simulink model "windTurbineSimulation"  (R2022a)
settings: Solver=FixedStepAuto  StartTime=0.0  StopTime=1000  FixedStep=0.001  RelTol=1e-3
libraries: embmathops x3
settings Model: Creator=S3945888  LastModifiedBy=119617
settings DebuggingCC: UnconnectedInputMsg=warning  UnconnectedOutputMsg=warning  UnconnectedLineMsg=warning
settings RTWCC: DLArmComputeVersion=19.05

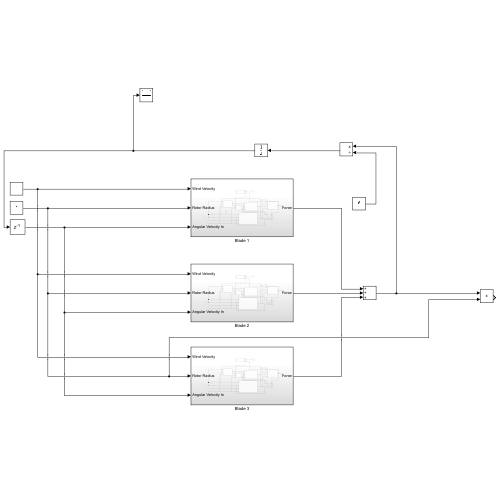
[thumbnail: Simulink's stored preview of the top-level diagram]
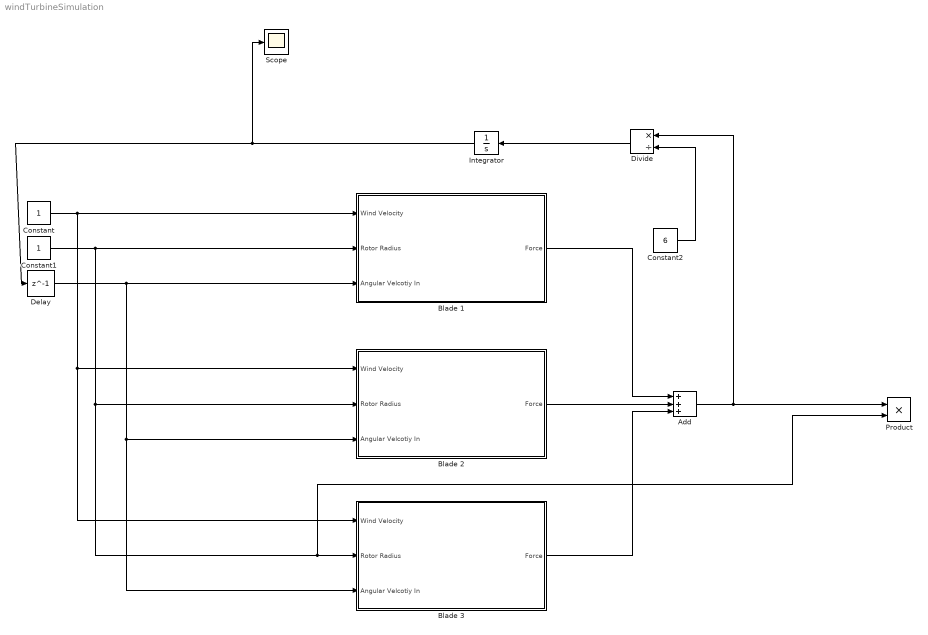
== system windTurbineSimulation ==
  Add : Sum  Inputs=+++
  Blade 1 : Subsystem
  Blade 2 : Subsystem
  Blade 3 : Subsystem
  Constant : Constant
  Constant1 : Constant
  Constant2 : Constant  Value=6
  Delay : Delay  DelayLength=1  InitialCondition=-6
  Divide : Product  Inputs=*/
  Integrator : Integrator  InitialCondition=-6
  Product : Product
  Scope : Scope
  wires:
  Constant/1 -> Blade 3/1(Wind Velocity), Blade 2/1(Wind Velocity), Blade 1/1(Wind Velocity)
  Constant1/1 -> Product/2, Blade 3/2(Rotor Radius), Blade 2/2(Rotor Radius), Blade 1/2(Rotor Radius)
  Blade 1/1(Force) -> Add/1
  Blade 2/1(Force) -> Add/2
  Blade 3/1(Force) -> Add/3
  Add/1 -> Divide/1, Product/1
  Delay/1 -> Blade 1/3(Angular Velcotiy In), Blade 3/3(Angular Velcotiy In), Blade 2/3(Angular Velcotiy In)
  Constant2/1 -> Divide/2
  Divide/1 -> Integrator/1
  Integrator/1 -> Scope/1, Delay/1

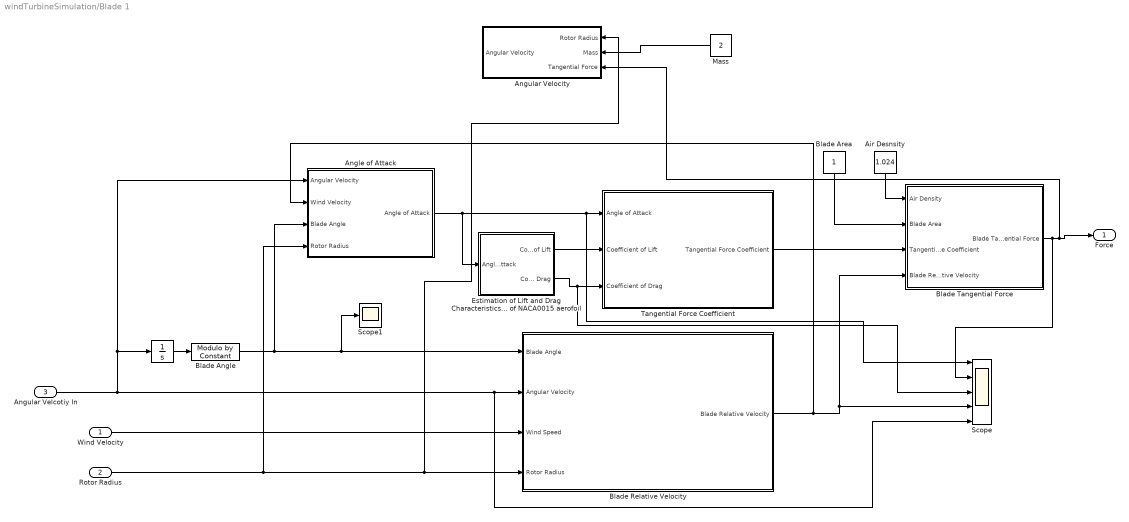
== system windTurbineSimulation/Blade 1 ==
  Wind Velocity : Inport
  Rotor Radius : Inport  Port=2
  Angular Velcotiy In : Inport  Port=3
  " " : Integrator
  Air Desnsity : Constant  Value=1.024
  Angle of Attack : Subsystem
  Angular Velocity : Subsystem
  Blade Angle : embmathops/Modulo by Constant  Denominator=2*pi  SimulateUsing=Code generation
      settings: SourceProductBaseCode=SL
  Blade Area : Constant
  Blade Relative Velocity : Subsystem
  Blade Tangential Force : Subsystem
  Estimation of Lift and Drag Characteristics of NACA0015 aerofoil : Subsystem
  Mass : Constant  Value=2
  Scope : Scope  NumInputPorts=5
  Scope1 : Scope
  Tangential Force Coefficient : Subsystem
  Force : Outport
  wires:
  Angular Velcotiy In/1 -> Angle of Attack/1(Angular Velocity), " "/1, Scope/5, Blade Relative Velocity/2(Angular Velocity)
  Air Desnsity/1 -> Blade Tangential Force/1(Air Density)
  Estimation of Lift and Drag Characteristics of NACA0015 aerofoil/2(Coefficient of Drag) -> Scope/3, Tangential Force Coefficient/3(Coefficient of Drag)
  Blade Angle/1 -> Angle of Attack/3(Blade Angle), Scope1/1, Blade Relative Velocity/1(Blade Angle)
  Tangential Force Coefficient/1(Tangential Force Coefficient) -> Blade Tangential Force/3(Tangential Force Coefficient)
  Angle of Attack/1(Angle of Attack) -> Scope/1, Tangential Force Coefficient/1(Angle of Attack), Estimation of Lift and Drag Characteristics of NACA0015 aerofoil/1(Angle of Attack)
  Blade Relative Velocity/1(Blade Relative Velocity) -> Angle of Attack/2(Wind Velocity), Scope/4, Blade Tangential Force/4(Blade Relative Velocity)
  Wind Velocity/1 -> Blade Relative Velocity/3(Wind Speed)
  Blade Tangential Force/1(Blade Tangential Force) -> Scope/2, Force/1, Angular Velocity/3(Tangential Force)
  Estimation of Lift and Drag Characteristics of NACA0015 aerofoil/1(Coefficient of Lift) -> Tangential Force Coefficient/2(Coefficient of Lift)
  Blade Area/1 -> Blade Tangential Force/2("Blade Area ")
  Mass/1 -> Angular Velocity/2(Mass)
  Rotor Radius/1 -> Angle of Attack/4(Rotor Radius), Angular Velocity/1(Rotor Radius), Blade Relative Velocity/4(Rotor Radius)
  " "/1 -> Blade Angle/1

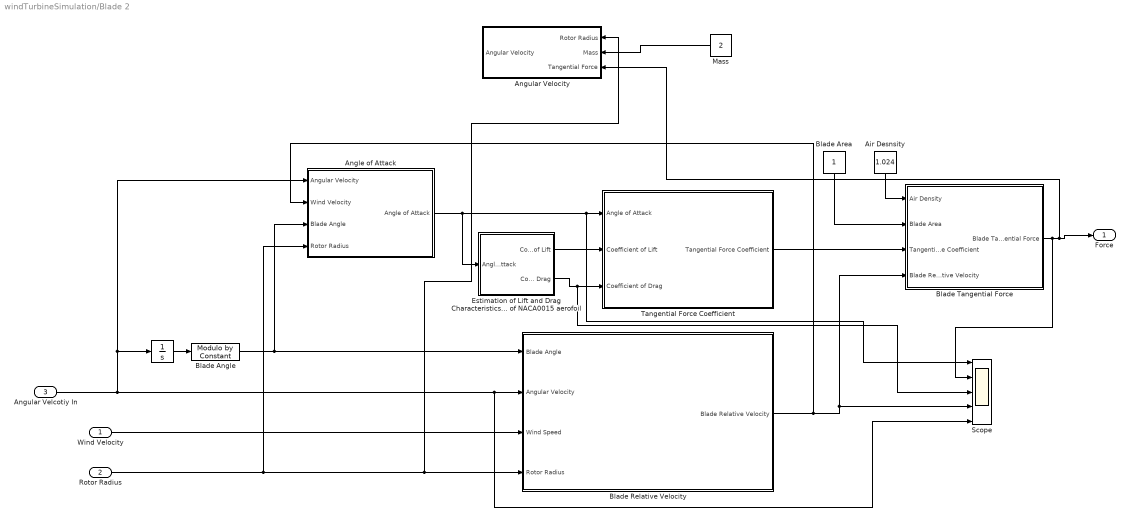
== system windTurbineSimulation/Blade 2 ==
  Wind Velocity : Inport
  Rotor Radius : Inport  Port=2
  Angular Velcotiy In : Inport  Port=3
  " " : Integrator
  Air Desnsity : Constant  Value=1.024
  Angle of Attack : Subsystem
  Angular Velocity : Subsystem
  Blade Angle : embmathops/Modulo by Constant  Denominator=2*pi  SimulateUsing=Code generation
      settings: SourceProductBaseCode=SL
  Blade Area : Constant
  Blade Relative Velocity : Subsystem
  Blade Tangential Force : Subsystem
  Estimation of Lift and Drag Characteristics of NACA0015 aerofoil : Subsystem
  Mass : Constant  Value=2
  Scope : Scope  NumInputPorts=5
  Tangential Force Coefficient : Subsystem
  Force : Outport
  wires:
  Angular Velcotiy In/1 -> Angle of Attack/1(Angular Velocity), " "/1, Scope/5, Blade Relative Velocity/2(Angular Velocity)
  Air Desnsity/1 -> Blade Tangential Force/1(Air Density)
  Estimation of Lift and Drag Characteristics of NACA0015 aerofoil/2(Coefficient of Drag) -> Scope/3, Tangential Force Coefficient/3(Coefficient of Drag)
  Blade Angle/1 -> Angle of Attack/3(Blade Angle), Blade Relative Velocity/1(Blade Angle)
  Tangential Force Coefficient/1(Tangential Force Coefficient) -> Blade Tangential Force/3(Tangential Force Coefficient)
  Angle of Attack/1(Angle of Attack) -> Scope/1, Tangential Force Coefficient/1(Angle of Attack), Estimation of Lift and Drag Characteristics of NACA0015 aerofoil/1(Angle of Attack)
  Blade Relative Velocity/1(Blade Relative Velocity) -> Angle of Attack/2(Wind Velocity), Scope/4, Blade Tangential Force/4(Blade Relative Velocity)
  Wind Velocity/1 -> Blade Relative Velocity/3(Wind Speed)
  Blade Tangential Force/1(Blade Tangential Force) -> Scope/2, Force/1, Angular Velocity/3(Tangential Force)
  Estimation of Lift and Drag Characteristics of NACA0015 aerofoil/1(Coefficient of Lift) -> Tangential Force Coefficient/2(Coefficient of Lift)
  Blade Area/1 -> Blade Tangential Force/2("Blade Area ")
  Mass/1 -> Angular Velocity/2(Mass)
  Rotor Radius/1 -> Angle of Attack/4(Rotor Radius), Angular Velocity/1(Rotor Radius), Blade Relative Velocity/4(Rotor Radius)
  " "/1 -> Blade Angle/1

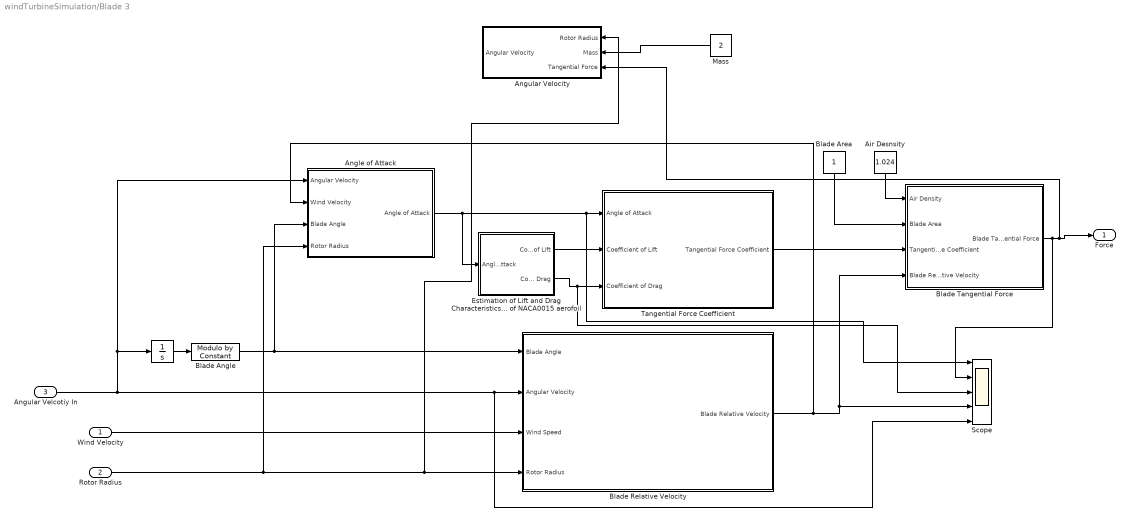
== system windTurbineSimulation/Blade 3 ==
  Wind Velocity : Inport
  Rotor Radius : Inport  Port=2
  Angular Velcotiy In : Inport  Port=3
  " " : Integrator
  Air Desnsity : Constant  Value=1.024
  Angle of Attack : Subsystem
  Angular Velocity : Subsystem
  Blade Angle : embmathops/Modulo by Constant  Denominator=2*pi  SimulateUsing=Code generation
      settings: SourceProductBaseCode=SL
  Blade Area : Constant
  Blade Relative Velocity : Subsystem
  Blade Tangential Force : Subsystem
  Estimation of Lift and Drag Characteristics of NACA0015 aerofoil : Subsystem
  Mass : Constant  Value=2
  Scope : Scope  NumInputPorts=5
  Tangential Force Coefficient : Subsystem
  Force : Outport
  wires:
  Angular Velcotiy In/1 -> Angle of Attack/1(Angular Velocity), " "/1, Scope/5, Blade Relative Velocity/2(Angular Velocity)
  Air Desnsity/1 -> Blade Tangential Force/1(Air Density)
  Estimation of Lift and Drag Characteristics of NACA0015 aerofoil/2(Coefficient of Drag) -> Scope/3, Tangential Force Coefficient/3(Coefficient of Drag)
  Blade Angle/1 -> Angle of Attack/3(Blade Angle), Blade Relative Velocity/1(Blade Angle)
  Tangential Force Coefficient/1(Tangential Force Coefficient) -> Blade Tangential Force/3(Tangential Force Coefficient)
  Angle of Attack/1(Angle of Attack) -> Scope/1, Tangential Force Coefficient/1(Angle of Attack), Estimation of Lift and Drag Characteristics of NACA0015 aerofoil/1(Angle of Attack)
  Blade Relative Velocity/1(Blade Relative Velocity) -> Angle of Attack/2(Wind Velocity), Scope/4, Blade Tangential Force/4(Blade Relative Velocity)
  Wind Velocity/1 -> Blade Relative Velocity/3(Wind Speed)
  Blade Tangential Force/1(Blade Tangential Force) -> Scope/2, Force/1, Angular Velocity/3(Tangential Force)
  Estimation of Lift and Drag Characteristics of NACA0015 aerofoil/1(Coefficient of Lift) -> Tangential Force Coefficient/2(Coefficient of Lift)
  Blade Area/1 -> Blade Tangential Force/2("Blade Area ")
  Mass/1 -> Angular Velocity/2(Mass)
  Rotor Radius/1 -> Angle of Attack/4(Rotor Radius), Angular Velocity/1(Rotor Radius), Blade Relative Velocity/4(Rotor Radius)
  " "/1 -> Blade Angle/1

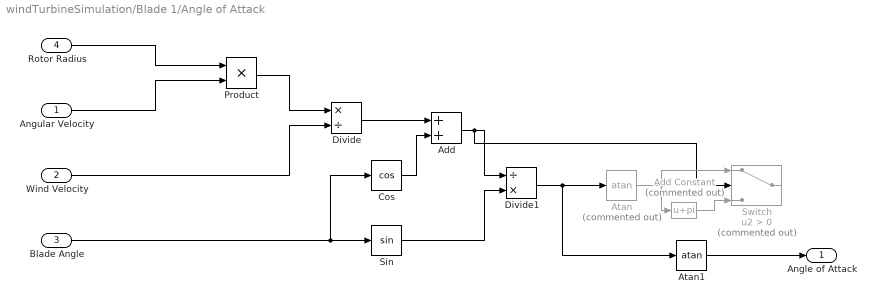
== system windTurbineSimulation/Blade 1/Angle of Attack ==
  Angular Velocity : Inport
  Wind Velocity : Inport  Port=2
  Blade Angle : Inport  Port=3
  Rotor Radius : Inport  Port=4
  Add : Sum
  Add Constant : Bias  Commented=on  Bias=pi  SaturateOnIntegerOverflow=off
  Atan : Trigonometry  Commented=on  Operator=atan
  Atan1 : Trigonometry  Operator=atan
  Cos : Trigonometry  Operator=cos
  Divide : Product  Inputs=*/
  Divide1 : Product  Inputs=/*
  Product : Product
  Sin : Trigonometry
  Switch : Switch  Commented=on  Criteria=u2 > Threshold  SaturateOnIntegerOverflow=off  InputSameDT=off
  Angle of Attack : Outport
  wires:
  Angular Velocity/1 -> Product/2
  Rotor Radius/1 -> Product/1
  Wind Velocity/1 -> Divide/2
  Product/1 -> Divide/1
  Divide/1 -> Add/1
  Cos/1 -> Add/2
  Blade Angle/1 -> Sin/1, Cos/1
  Add/1 -> Switch/2, Divide1/1
  Sin/1 -> Divide1/2
  Divide1/1 -> Atan1/1, Atan/1
  Atan/1 -> Add Constant/1, Switch/1
  Add Constant/1 -> Switch/3
  Atan1/1 -> Angle of Attack/1

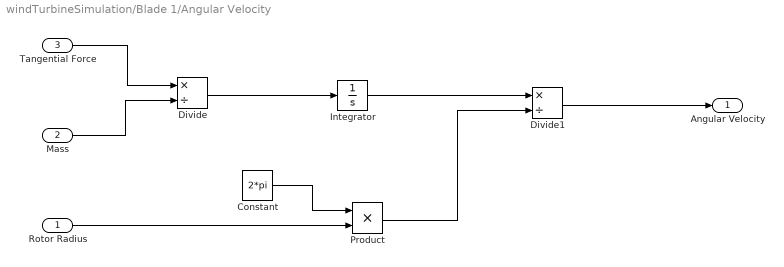
== system windTurbineSimulation/Blade 1/Angular Velocity ==
  Rotor Radius : Inport
  Mass : Inport  Port=2
  Tangential Force : Inport  Port=3
  Constant : Constant  Value=2*pi
  Divide : Product  Inputs=*/
  Divide1 : Product  Inputs=*/
  Integrator : Integrator
  Product : Product
  Angular Velocity : Outport
  wires:
  Mass/1 -> Divide/2
  Tangential Force/1 -> Divide/1
  Divide/1 -> Integrator/1
  Integrator/1 -> Divide1/1
  Rotor Radius/1 -> Product/2
  Constant/1 -> Product/1
  Product/1 -> Divide1/2
  Divide1/1 -> Angular Velocity/1

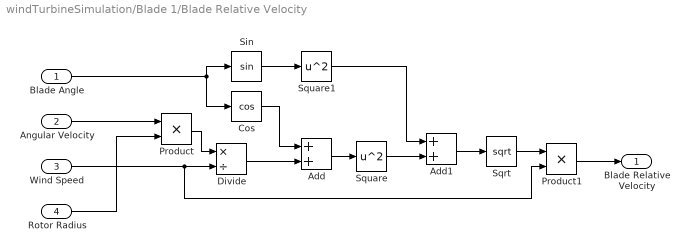
== system windTurbineSimulation/Blade 1/Blade Relative Velocity ==
  Blade Angle : Inport
  Angular Velocity : Inport  Port=2
  Wind Speed : Inport  Port=3
  Rotor Radius : Inport  Port=4
  Add : Sum
  Add1 : Sum
  Cos : Trigonometry  Operator=cos
  Divide : Product  Inputs=*/
  Product : Product
  Product1 : Product
  Sin : Trigonometry
  Sqrt : Sqrt
  Square : Math  Operator=square
  Square1 : Math  Operator=square
  Blade Relative Velocity : Outport
  wires:
  Angular Velocity/1 -> Product/1
  Square1/1 -> Add1/1
  Add1/1 -> Sqrt/1
  Square/1 -> Add1/2
  Product/1 -> Divide/1
  Wind Speed/1 -> Product1/2, Divide/2
  Divide/1 -> Add/2
  Sqrt/1 -> Product1/1
  Blade Angle/1 -> Cos/1, Sin/1
  Cos/1 -> Add/1
  Sin/1 -> Square1/1
  Add/1 -> Square/1
  Rotor Radius/1 -> Product/2
  Product1/1 -> Blade Relative Velocity/1

== system windTurbineSimulation/Blade 1/Blade Tangential Force ==
  Air Density : Inport
  "Blade Area " : Inport  Port=2
  Tangential Force Coefficient : Inport  Port=3
  Blade Relative Velocity : Inport  Port=4
  Gain : Gain  Gain=0.5
  Product : Product  Inputs=4
  Square : Math  Operator=square
  Blade Tangential Force : Outport
  wires:
  Blade Relative Velocity/1 -> Square/1
  Square/1 -> Product/4
  Tangential Force Coefficient/1 -> Product/3
  "Blade Area "/1 -> Product/2
  Air Density/1 -> Product/1
  Product/1 -> Gain/1
  Gain/1 -> Blade Tangential Force/1

== system windTurbineSimulation/Blade 1/Estimation of Lift and Drag Characteristics of NACA0015 aerofoil ==
  Angle of Attack : Inport
  Add Constant : Bias  Bias=1  SaturateOnIntegerOverflow=off
  Cos : Trigonometry  Operator=cos
  Gain : Gain  Gain=2
  Gain1 : Gain  Gain=-0.8
  Sin : Trigonometry
  Coefficient of Lift : Outport
  Coefficient of Drag : Outport  Port=2
  wires:
  Angle of Attack/1 -> Gain/1
  Gain/1 -> Cos/1, Sin/1
  Cos/1 -> Gain1/1
  Sin/1 -> Coefficient of Lift/1
  Gain1/1 -> Add Constant/1
  Add Constant/1 -> Coefficient of Drag/1

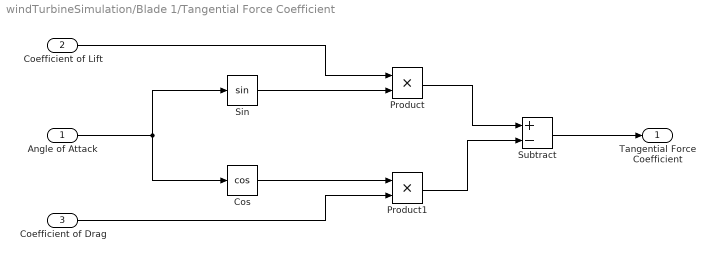
== system windTurbineSimulation/Blade 1/Tangential Force Coefficient ==
  Angle of Attack : Inport
  Coefficient of Lift : Inport  Port=2
  Coefficient of Drag : Inport  Port=3
  Cos : Trigonometry  Operator=cos
  Product : Product
  Product1 : Product
  Sin : Trigonometry
  Subtract : Sum  Inputs=+-
  Tangential Force Coefficient : Outport
  wires:
  Sin/1 -> Product/2
  Cos/1 -> Product1/1
  Angle of Attack/1 -> Cos/1, Sin/1
  Coefficient of Lift/1 -> Product/1
  Coefficient of Drag/1 -> Product1/2
  Subtract/1 -> Tangential Force Coefficient/1
  Product1/1 -> Subtract/2
  Product/1 -> Subtract/1

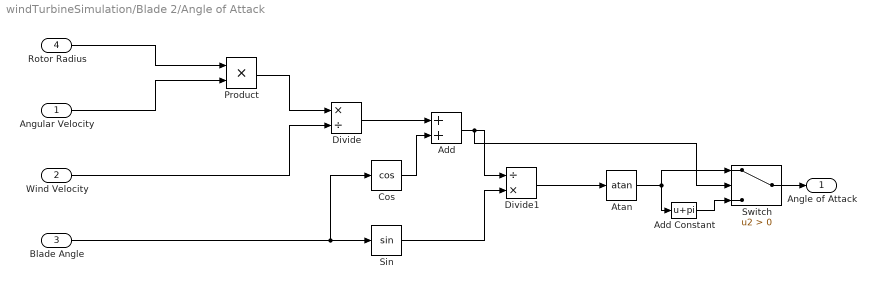
== system windTurbineSimulation/Blade 2/Angle of Attack ==
  Angular Velocity : Inport
  Wind Velocity : Inport  Port=2
  Blade Angle : Inport  Port=3
  Rotor Radius : Inport  Port=4
  Add : Sum
  Add Constant : Bias  Bias=pi  SaturateOnIntegerOverflow=off
  Atan : Trigonometry  Operator=atan
  Cos : Trigonometry  Operator=cos
  Divide : Product  Inputs=*/
  Divide1 : Product  Inputs=/*
  Product : Product
  Sin : Trigonometry
  Switch : Switch  Criteria=u2 > Threshold  SaturateOnIntegerOverflow=off  InputSameDT=off
  Angle of Attack : Outport
  wires:
  Angular Velocity/1 -> Product/2
  Rotor Radius/1 -> Product/1
  Wind Velocity/1 -> Divide/2
  Product/1 -> Divide/1
  Divide/1 -> Add/1
  Cos/1 -> Add/2
  Blade Angle/1 -> Sin/1, Cos/1
  Add/1 -> Switch/2, Divide1/1
  Sin/1 -> Divide1/2
  Divide1/1 -> Atan/1
  Switch/1 -> Angle of Attack/1
  Atan/1 -> Add Constant/1, Switch/1
  Add Constant/1 -> Switch/3

== system windTurbineSimulation/Blade 2/Angular Velocity ==
  Rotor Radius : Inport
  Mass : Inport  Port=2
  Tangential Force : Inport  Port=3
  Constant : Constant  Value=2*pi
  Divide : Product  Inputs=*/
  Divide1 : Product  Inputs=*/
  Integrator : Integrator
  Product : Product
  Angular Velocity : Outport
  wires:
  Mass/1 -> Divide/2
  Tangential Force/1 -> Divide/1
  Divide/1 -> Integrator/1
  Integrator/1 -> Divide1/1
  Rotor Radius/1 -> Product/2
  Constant/1 -> Product/1
  Product/1 -> Divide1/2
  Divide1/1 -> Angular Velocity/1

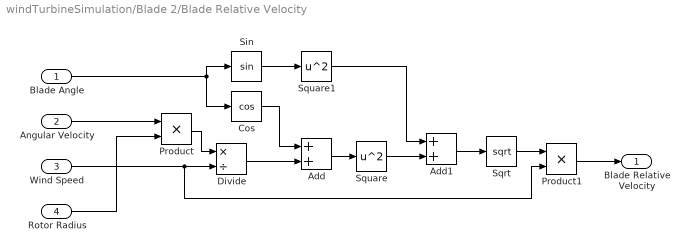
== system windTurbineSimulation/Blade 2/Blade Relative Velocity ==
  Blade Angle : Inport
  Angular Velocity : Inport  Port=2
  Wind Speed : Inport  Port=3
  Rotor Radius : Inport  Port=4
  Add : Sum
  Add1 : Sum
  Cos : Trigonometry  Operator=cos
  Divide : Product  Inputs=*/
  Product : Product
  Product1 : Product
  Sin : Trigonometry
  Sqrt : Sqrt
  Square : Math  Operator=square
  Square1 : Math  Operator=square
  Blade Relative Velocity : Outport
  wires:
  Angular Velocity/1 -> Product/1
  Square1/1 -> Add1/1
  Add1/1 -> Sqrt/1
  Square/1 -> Add1/2
  Product/1 -> Divide/1
  Wind Speed/1 -> Product1/2, Divide/2
  Divide/1 -> Add/2
  Sqrt/1 -> Product1/1
  Blade Angle/1 -> Cos/1, Sin/1
  Cos/1 -> Add/1
  Sin/1 -> Square1/1
  Add/1 -> Square/1
  Rotor Radius/1 -> Product/2
  Product1/1 -> Blade Relative Velocity/1

== system windTurbineSimulation/Blade 2/Blade Tangential Force ==
  Air Density : Inport
  "Blade Area " : Inport  Port=2
  Tangential Force Coefficient : Inport  Port=3
  Blade Relative Velocity : Inport  Port=4
  Gain : Gain  Gain=0.5
  Product : Product  Inputs=4
  Square : Math  Operator=square
  Blade Tangential Force : Outport
  wires:
  Blade Relative Velocity/1 -> Square/1
  Square/1 -> Product/4
  Tangential Force Coefficient/1 -> Product/3
  "Blade Area "/1 -> Product/2
  Air Density/1 -> Product/1
  Product/1 -> Gain/1
  Gain/1 -> Blade Tangential Force/1

== system windTurbineSimulation/Blade 2/Estimation of Lift and Drag Characteristics of NACA0015 aerofoil ==
  Angle of Attack : Inport
  Add Constant : Bias  Bias=1  SaturateOnIntegerOverflow=off
  Cos : Trigonometry  Operator=cos
  Gain : Gain  Gain=2
  Gain1 : Gain  Gain=-0.8
  Sin : Trigonometry
  Coefficient of Lift : Outport
  Coefficient of Drag : Outport  Port=2
  wires:
  Angle of Attack/1 -> Gain/1
  Gain/1 -> Cos/1, Sin/1
  Cos/1 -> Gain1/1
  Sin/1 -> Coefficient of Lift/1
  Gain1/1 -> Add Constant/1
  Add Constant/1 -> Coefficient of Drag/1

== system windTurbineSimulation/Blade 2/Tangential Force Coefficient ==
  Angle of Attack : Inport
  Coefficient of Lift : Inport  Port=2
  Coefficient of Drag : Inport  Port=3
  Cos : Trigonometry  Operator=cos
  Product : Product
  Product1 : Product
  Sin : Trigonometry
  Subtract : Sum  Inputs=+-
  Tangential Force Coefficient : Outport
  wires:
  Sin/1 -> Product/2
  Cos/1 -> Product1/1
  Angle of Attack/1 -> Cos/1, Sin/1
  Coefficient of Lift/1 -> Product/1
  Coefficient of Drag/1 -> Product1/2
  Subtract/1 -> Tangential Force Coefficient/1
  Product1/1 -> Subtract/2
  Product/1 -> Subtract/1

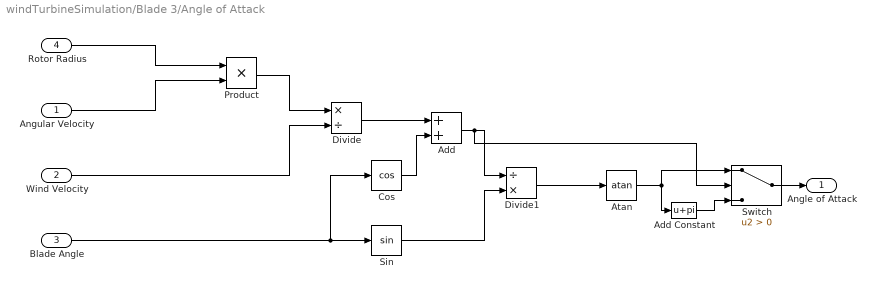
== system windTurbineSimulation/Blade 3/Angle of Attack ==
  Angular Velocity : Inport
  Wind Velocity : Inport  Port=2
  Blade Angle : Inport  Port=3
  Rotor Radius : Inport  Port=4
  Add : Sum
  Add Constant : Bias  Bias=pi  SaturateOnIntegerOverflow=off
  Atan : Trigonometry  Operator=atan
  Cos : Trigonometry  Operator=cos
  Divide : Product  Inputs=*/
  Divide1 : Product  Inputs=/*
  Product : Product
  Sin : Trigonometry
  Switch : Switch  Criteria=u2 > Threshold  SaturateOnIntegerOverflow=off  InputSameDT=off
  Angle of Attack : Outport
  wires:
  Angular Velocity/1 -> Product/2
  Rotor Radius/1 -> Product/1
  Wind Velocity/1 -> Divide/2
  Product/1 -> Divide/1
  Divide/1 -> Add/1
  Cos/1 -> Add/2
  Blade Angle/1 -> Sin/1, Cos/1
  Add/1 -> Switch/2, Divide1/1
  Sin/1 -> Divide1/2
  Divide1/1 -> Atan/1
  Switch/1 -> Angle of Attack/1
  Atan/1 -> Add Constant/1, Switch/1
  Add Constant/1 -> Switch/3

== system windTurbineSimulation/Blade 3/Angular Velocity ==
  Rotor Radius : Inport
  Mass : Inport  Port=2
  Tangential Force : Inport  Port=3
  Constant : Constant  Value=2*pi
  Divide : Product  Inputs=*/
  Divide1 : Product  Inputs=*/
  Integrator : Integrator
  Product : Product
  Angular Velocity : Outport
  wires:
  Mass/1 -> Divide/2
  Tangential Force/1 -> Divide/1
  Divide/1 -> Integrator/1
  Integrator/1 -> Divide1/1
  Rotor Radius/1 -> Product/2
  Constant/1 -> Product/1
  Product/1 -> Divide1/2
  Divide1/1 -> Angular Velocity/1

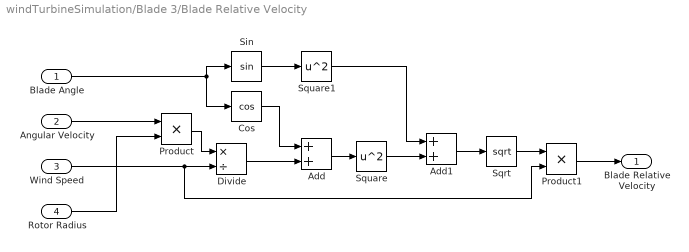
== system windTurbineSimulation/Blade 3/Blade Relative Velocity ==
  Blade Angle : Inport
  Angular Velocity : Inport  Port=2
  Wind Speed : Inport  Port=3
  Rotor Radius : Inport  Port=4
  Add : Sum
  Add1 : Sum
  Cos : Trigonometry  Operator=cos
  Divide : Product  Inputs=*/
  Product : Product
  Product1 : Product
  Sin : Trigonometry
  Sqrt : Sqrt
  Square : Math  Operator=square
  Square1 : Math  Operator=square
  Blade Relative Velocity : Outport
  wires:
  Angular Velocity/1 -> Product/1
  Square1/1 -> Add1/1
  Add1/1 -> Sqrt/1
  Square/1 -> Add1/2
  Product/1 -> Divide/1
  Wind Speed/1 -> Product1/2, Divide/2
  Divide/1 -> Add/2
  Sqrt/1 -> Product1/1
  Blade Angle/1 -> Cos/1, Sin/1
  Cos/1 -> Add/1
  Sin/1 -> Square1/1
  Add/1 -> Square/1
  Rotor Radius/1 -> Product/2
  Product1/1 -> Blade Relative Velocity/1

== system windTurbineSimulation/Blade 3/Blade Tangential Force ==
  Air Density : Inport
  "Blade Area " : Inport  Port=2
  Tangential Force Coefficient : Inport  Port=3
  Blade Relative Velocity : Inport  Port=4
  Gain : Gain  Gain=0.5
  Product : Product  Inputs=4
  Square : Math  Operator=square
  Blade Tangential Force : Outport
  wires:
  Blade Relative Velocity/1 -> Square/1
  Square/1 -> Product/4
  Tangential Force Coefficient/1 -> Product/3
  "Blade Area "/1 -> Product/2
  Air Density/1 -> Product/1
  Product/1 -> Gain/1
  Gain/1 -> Blade Tangential Force/1

== system windTurbineSimulation/Blade 3/Estimation of Lift and Drag Characteristics of NACA0015 aerofoil ==
  Angle of Attack : Inport
  Add Constant : Bias  Bias=1  SaturateOnIntegerOverflow=off
  Cos : Trigonometry  Operator=cos
  Gain : Gain  Gain=2
  Gain1 : Gain  Gain=-0.8
  Sin : Trigonometry
  Coefficient of Lift : Outport
  Coefficient of Drag : Outport  Port=2
  wires:
  Angle of Attack/1 -> Gain/1
  Gain/1 -> Cos/1, Sin/1
  Cos/1 -> Gain1/1
  Sin/1 -> Coefficient of Lift/1
  Gain1/1 -> Add Constant/1
  Add Constant/1 -> Coefficient of Drag/1

== system windTurbineSimulation/Blade 3/Tangential Force Coefficient ==
  Angle of Attack : Inport
  Coefficient of Lift : Inport  Port=2
  Coefficient of Drag : Inport  Port=3
  Cos : Trigonometry  Operator=cos
  Product : Product
  Product1 : Product
  Sin : Trigonometry
  Subtract : Sum  Inputs=+-
  Tangential Force Coefficient : Outport
  wires:
  Sin/1 -> Product/2
  Cos/1 -> Product1/1
  Angle of Attack/1 -> Cos/1, Sin/1
  Coefficient of Lift/1 -> Product/1
  Coefficient of Drag/1 -> Product1/2
  Subtract/1 -> Tangential Force Coefficient/1
  Product1/1 -> Subtract/2
  Product/1 -> Subtract/1
